simulink model "myexp7"  (R2022a)
settings: Solver=VariableStepAuto  StartTime=0.0  StopTime=10  RelTol=1e-3
libraries: dspstat3 x4, commchan3 x1, commrandsrc3 x1, commsink2 x1, commfilt2 x1, dspsigops x1
settings Model: Creator=惠普  LastModifiedBy=惠普

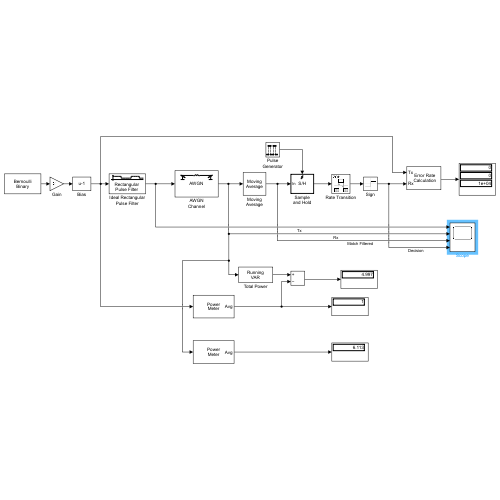
[thumbnail: Simulink's stored preview of the top-level diagram]
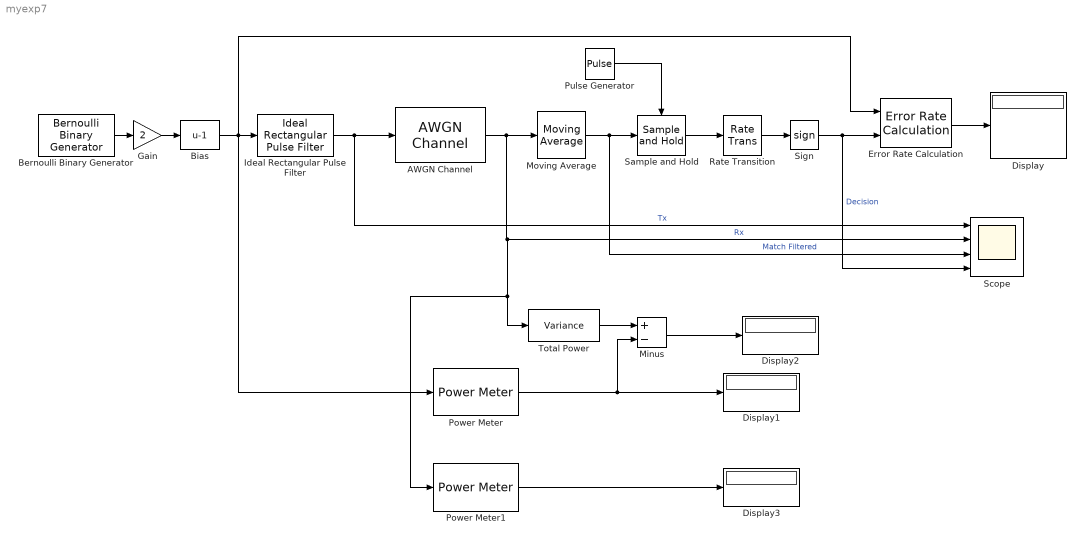
== system myexp7 ==
  AWGN Channel : commchan3/AWGN Channel  InputProcessing=Columns as channels (frame based)  seed=137  noiseMode="Signal to noise ratio  (Es/No)"  EbNodB=10  EsNodB=10  SNRdB=10  bitsPerSym=1  Ps=1  Tsym=1e-3  variance=1
  Bernoulli Binary Generator : commrandsrc3/Bernoulli Binary Generator  ProbabilityOfZero=0.5  SeedSource=Auto  Seed=0  SampleTime=1e-3  SamplesPerFrame=1  OutputDataType=double  SimulateUsing=Interpreted execution
  Bias : Bias  Bias=-1  SaturateOnIntegerOverflow=off
  Display{,1..3} (4 alike) : Display
  Error Rate Calculation : commsink2/Error Rate Calculation  N=1  st_delay=0  cp_mode=Entire frame  subframe=[]  PMode=Port  WsName=ErrorVec  RsMode2=off  stop=off  numErr=100  maxBits=1e6
  Gain : Gain  Gain=2
  Ideal Rectangular Pulse Filter : commfilt2/Ideal Rectangular Pulse Filter  pulseLen=100  pulseDelay=0  InputProcessing=Columns as channels (frame based)  RateOptions=Allow multirate processing  sampMode=Mute  normCheck=off  normMode=Sum of samples  filterGain=1  saveAsFlag=0  roundingMode=Floor  overflowMode=off  firstCoeffDataTypeStr=Inherit: Same word length as input  firstCoeffMin=[]  firstCoeffMax=[]  firstCoeffLastDataTypeStr=Inherit: Same word length as input  outputDataTypeStr=Inherit: Same as accumulator  outputMin=[]  outputMax=[]  outputLastDataTypeStr=Inherit: Same as accumulator
      settings: SourceProductBaseCode=CM
  Minus : Sum  Inputs=+-
  Moving Average : dspstat3/Moving Average  Method=Sliding window  ForgettingFactorPort=off  SpecifyWindowLength=on  WindowLength=100  ForgettingFactor=0.9  SimulateUsing=Code generation
  Power Meter : dspstat3/Power Meter  Measurement=Average power  WindowLength=500  ReferenceLoad=1  OutputPowerUnits=Watts  SimulateUsing=Code generation
      settings: SourceProductBaseCode=DS
  Power Meter1 : dspstat3/Power Meter  Measurement=Average power  WindowLength=1000  ReferenceLoad=1  OutputPowerUnits=Watts  SimulateUsing=Code generation
      settings: SourceProductBaseCode=DS
  Pulse Generator : DiscretePulseGenerator  Period=100  SampleTime=10e-6
  Rate Transition : RateTransition  OutPortSampleTime=1e-3
  Sample and Hold : dspsigops/Sample and Hold  trig=Rising edge  initCond=0  latchinput=off
  Scope : Scope  NumInputPorts=4
  Sign : Signum
  Total Power : dspstat3/Variance  run=on  InputProcessing=Columns as channels (frame based)  reset_popup=None  directionMode=Each column  dimension=1  roiEnable=off  roiType=Rectangles  roiPortion=Entire ROI  roiOutput=Individual statistics for each ROI  roiFlag=off  roundingMode=Floor  overflowMode=off
  wires:
  Bernoulli Binary Generator/1 -> Gain/1
  Gain/1 -> Bias/1
  Bias/1 -> Power Meter/1, Error Rate Calculation/1, Ideal Rectangular Pulse Filter/1
  Ideal Rectangular Pulse Filter/1 -> Scope/1, AWGN Channel/1  "Tx"
  AWGN Channel/1 -> Power Meter1/1, Total Power/1, Scope/2, Moving Average/1  "Rx"
  Moving Average/1 -> Scope/3, Sample and Hold/1  "Match Filtered"
  Pulse Generator/1 -> Sample and Hold/Trigger
  Sample and Hold/1 -> Rate Transition/1
  Rate Transition/1 -> Sign/1
  Sign/1 -> Scope/4, Error Rate Calculation/2  "Decision"
  Error Rate Calculation/1 -> Display/1
  Power Meter/1 -> Minus/2, Display1/1
  Total Power/1 -> Minus/1
  Minus/1 -> Display2/1
  Power Meter1/1 -> Display3/1
